simulink model "FACTORIAL"  (R2021a)
settings: Solver=VariableStepAuto  StartTime=0.0  StopTime=10.0  RelTol=1e-3
settings Model: Creator=Osman  LastModifiedBy=Osman

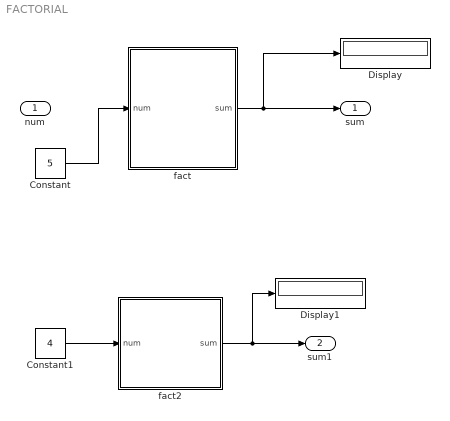
== system FACTORIAL ==
  num : Inport
  Constant : Constant  Value=5  OutDataTypeStr=uint32
  Constant1 : Constant  Value=4  OutDataTypeStr=uint32
  Display : Display
  Display1 : Display
  fact : Stateflow chart  TreatAsAtomicUnit=on
  fact2 : Stateflow chart  TreatAsAtomicUnit=on
  sum : Outport
  sum1 : Outport  Port=2
  wires:
  fact/1(sum) -> Display/1, sum/1
  Constant/1 -> fact/1(num)
  Constant1/1 -> fact2/1(num)
  fact2/1(sum) -> Display1/1, sum1/1

== stateflow chart FACTORIAL/fact2 ==
  state init
    entry:
    i = 1;
    sum = 1;
  state calc
    entry:
    sum = sum * i;
    i = i +1;
  (default) -> init
  init -> calc
  calc -> calc : [i <= num]
  data: i local uint32; sum output uint32; num input uint32

== stateflow chart FACTORIAL/fact ==
  (default) -> (junction 8) : % fact
  (junction 8) -> (junction 10) : {i = 1; sum = 1;}
  (junction 10) -> (junction 9) [order 1] : [i <= num]
  (junction 9) -> (junction 11) : {sum = sum * i;}
  (junction 12) -> (junction 10)
  (junction 10) -> (junction 13) [order 2]
  (junction 11) -> (junction 12) : {i = i +1;}
  data: i local uint32; num input uint32; sum output uint32
